simulink model "mli9lvlhbrd"  (Simulink 7.9)
settings: Solver=ode45  StartTime=0.0  StopTime=1  RelTol=1e-3
libraries: powerlib x13, simulink x4
settings Model: Creator=DILEEP KUMAR  LastModifiedBy=DILEEP KUMAR

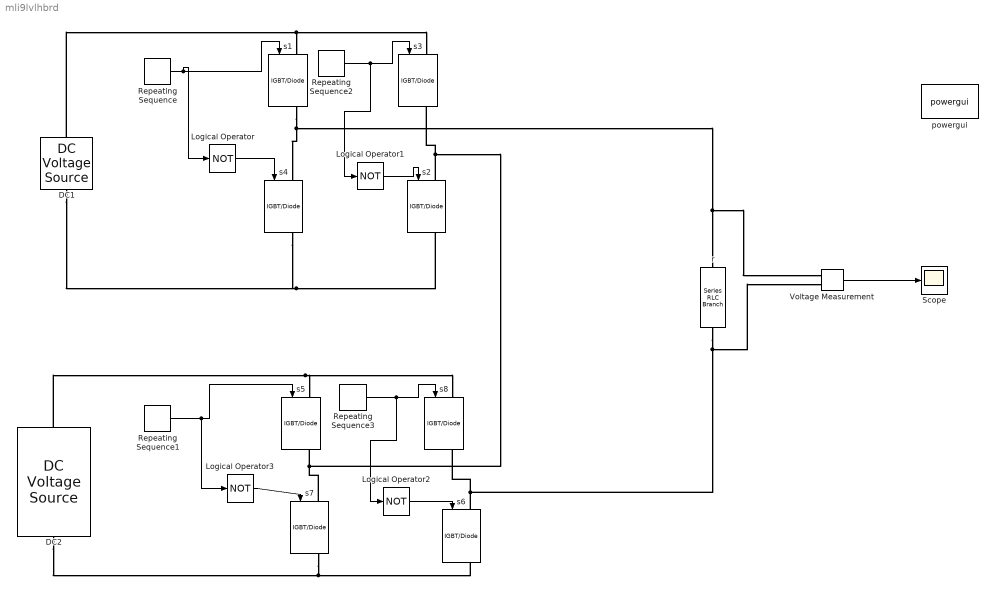
== system mli9lvlhbrd ==
  DC1 : powerlib/Electrical Sources/DC Voltage Source  Amplitude=100  Measurements=None
  DC2 : powerlib/Electrical Sources/DC Voltage Source  Amplitude=300  Measurements=None
  Logical Operator{,1..3} (4 alike) : Logic  Operator=NOT  AllPortsSameDT=off  OutDataTypeStr=boolean
  Repeating Sequence : simulink/Sources/Repeating Sequence  rep_seq_t=[0 1 1 2 2 4 4 6 6 8 8 9 9 11 11 12 12 16 16 17 17 18]*(0.02/18)  rep_seq_y=[0 0 1 1 0 0 1 1 0 0 1 1 0 0 1 1 0 0 1 1 0 0]
  Repeating Sequence1 : simulink/Sources/Repeating Sequence  rep_seq_t=[0 2 2 8 8 18]*(0.02/18)  rep_seq_y=[0 0 1 1 0 0]
  Repeating Sequence2 : simulink/Sources/Repeating Sequence  rep_seq_t=[0 2 2 3 3 7 7 8 8 10 10 11 11 13 13 15 15 17 17 18 18]*(0.02/18)  rep_seq_y=[0 0 1 1 0 0 1 1 0 0 1 1 0 0 1 1 0 0 1 1 0]
  Repeating Sequence3 : simulink/Sources/Repeating Sequence  rep_seq_t=[0 11 11 17 17 18]*(0.02/18)  rep_seq_y=[0 0 1 1 0 0]
  Scope : Scope
      settings: SaveName=reductionh
  Voltage Measurement : powerlib/Measurements/Voltage Measurement  PhasorSimulation=off  OutputType=Complex  PSBequivalent=0
  powergui : powerlib/powergui  Priority=1  SimulationMode=Discrete  SolverType=Tustin  SampleTime=50e-6  frequency=60  SPID=off  DisableSnubberDevices=off  DisableRonSwitches=off  DisableVfSwitches=off  SwTol=0  Interpol=off  DisplayEquations=off  FunctionMessages=off  frequencyindice=0  Pbase=100e6  ErrMax=1e-4  Iterations=50  UnitsV=kV  UnitsW=MW  echomessages=off  HookPort=off  EnableUseOfTLC=off  x0status=blocks  RestoreLinks=warning  ResistiveCurrentMeasurement=off  Ylog=off  Xlog=on  ShowGrid=off  save=off  variable=ZData  structure=reductionh  ZoomFFT=off  StartTime=0.2  cycles=1  DisplayStyle=1  fundamental=50  FreqAxis=off  MaxFrequency=1000  frequencyindicesteady=1  display=off  methode=off
  r : powerlib/Elements/Series RLC Branch  LConnTagsString=__new0  RConnTagsString=__new0  BranchType=R  Resistance=10  Inductance=1e-3  SetiL0=off  InitialCurrent=0  Capacitance=1e-6  Setx0=off  InitialVoltage=0  Measurements=None
  s{1..8} (8 alike) : powerlib/Power Electronics/IGBT//Diode  Ron=1e-3  Rs=1e5  Cs=inf  Measurements=on
  wires:
  Repeating Sequence/1 -> s1/1, Logical Operator/1
  Repeating Sequence2/1 -> s3/1, Logical Operator1/1
  Voltage Measurement/1 -> Scope/1
  Logical Operator/1 -> s4/1
  Logical Operator1/1 -> s2/1
  Repeating Sequence1/1 -> s5/1, Logical Operator3/1
  Repeating Sequence3/1 -> s8/1, Logical Operator2/1
  Logical Operator2/1 -> s6/1
  Logical Operator3/1 -> s7/1
  connections:
  DC1/RConn1 -- s3/LConn1 -- s1/LConn1
  s1/RConn1 -- s4/LConn1 -- r/LConn1 -- Voltage Measurement/LConn1
  DC1/LConn1 -- s2/RConn1 -- s4/RConn1
  s2/LConn1 -- s3/RConn1 -- s7/LConn1 -- s5/RConn1
  r/RConn1 -- Voltage Measurement/LConn2 -- s6/LConn1 -- s8/RConn1
  DC2/RConn1 -- s8/LConn1 -- s5/LConn1
  DC2/LConn1 -- s6/RConn1 -- s7/RConn1
